simulink model "vehicle_sim"  (R2018b)
settings: Solver=VariableStepAuto  StartTime=0.0  StopTime=10.0  RelTol=1e-3
values from neighbouring files (symbols this model uses):
  delta_step = dmax/15    (= 0.0407243492132)    [vehicle_sim_main.m]
  Td_step = Tdmax/2.5    (= 353.3586)    [vehicle_sim_main.m]
  th = [m;Jz;a;b;Cf;Cr;rw;mu;Af;Al;Cx;Rr;rho]    [Parameters.m]    (also in vehicle_sim_main.m = [m;Jz;a;b;Cf;Cr;rw;mu;Tdmax;Tdmin;dmax;dmin;Af;Al;Cx;Rr;rho])
  Ts_slk = 1e-1    (= 0.1)    [vehicle_sim_main.m]
  xi0 = [X Y Ux beta psi r]'    [Vehicle_Project_Main.m]    (also in Vehicle_Project_Main_Edo.m; Vehicle_Project_Main_torque.m; initial_guess_setting.m; nonchiude.mat = [1.99964684616 -50.0000753453 20 0 -7.1628861126e-05 0])
settings Model: Creator=Lorenzo  LastModifiedBy=Lorenzo

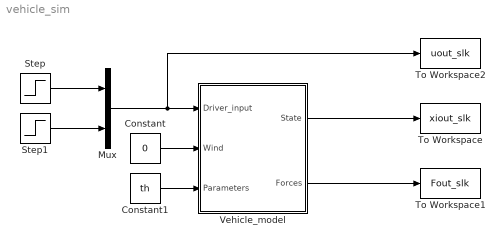
== system vehicle_sim ==
  Constant : Constant  Value=0
  Constant1 : Constant  Value=th
  Mux : Mux  Inputs=2
  Step : Step  Time=0  After=Td_step  SampleTime=0
  Step1 : Step  Time=0  After=delta_step  SampleTime=0
  To Workspace : ToWorkspace  VariableName=xiout_slk  SaveFormat=Structure With Time  SampleTime=Ts_slk
  To Workspace1 : ToWorkspace  VariableName=Fout_slk  SaveFormat=Structure With Time  SampleTime=Ts_slk
  To Workspace2 : ToWorkspace  VariableName=uout_slk  SaveFormat=Structure With Time  SampleTime=Ts_slk
  Vehicle_model : Subsystem
  wires:
  Vehicle_model/1(State) -> To Workspace/1
  Vehicle_model/2(Forces) -> To Workspace1/1
  Step/1 -> Mux/1
  Step1/1 -> Mux/2
  Mux/1 -> To Workspace2/1, Vehicle_model/1(Driver_input)
  Constant/1 -> Vehicle_model/2(Wind)
  Constant1/1 -> Vehicle_model/3(Parameters)

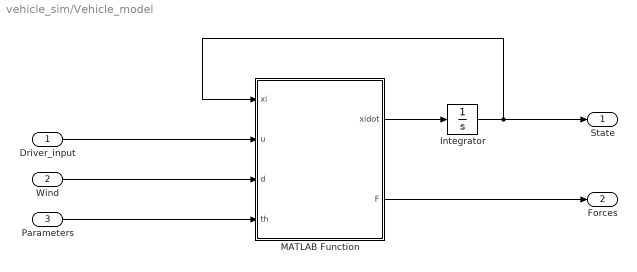
== system vehicle_sim/Vehicle_model ==
  Driver_input : Inport
  Wind : Inport  Port=2
  Parameters : Inport  Port=3
  Integrator : Integrator  InitialCondition=xi0
  MATLAB Function : MATLAB Function  TreatAsAtomicUnit=on
  State : Outport
  Forces : Outport  Port=2
  wires:
  Parameters/1 -> MATLAB Function/4(th)
  Integrator/1 -> State/1, MATLAB Function/1(xi)
  Wind/1 -> MATLAB Function/3(d)
  MATLAB Function/1(xidot) -> Integrator/1
  Driver_input/1 -> MATLAB Function/2(u)
  MATLAB Function/2(F) -> Forces/1

== matlab function vehicle_sim/Vehicle_model/MATLAB Function ==
  data: xi input; u input; xidot output; d input; th input; F output
function [xidot,F]=vehicle_model(xi,u,d,th)
% Nonlinear dynamic model of a road vehicle with six states: 2-D position,
% 2-D velocity, yaw angle and yaw rate. Nonlinear lateral tyre forces with
% Fiala model; saturation on braking and driving torque, saturation on 
% front wheel steering angle. Partial de-coupling of longitudinal and
% lateral dynamics (assume longitudinal speed varies slowly with respect to
% lateral dynamics)
%
% Inputs:   xi      (model state)
%           u       (braking/driving torque and steering angle)
%           d       (lateral wind),
%           
%           th      (model parameters)
%
% Outputs:  xi_dot  (derivative of the state with respect to time)
%           F       (longitudinal and lateral forces)

%% Read parameters, states and inputs
% Parameters
m       =       th(1,1);     % vehicle mass (kg)
Jz      =       th(2,1);     % vehicle moment of inertia (kg*m^2)
a       =       th(3,1);     % distance between center of gravity and front axle (m)
b       =       th(4,1);     % distance between center of gravity and rear axle (m)
Cf      =       th(5,1);     % front axle cornering stiffness (N/rad)
Cr      =       th(6,1);     % rear axle cornering stiffness (N/rad)
rw      =       th(7,1);     % wheel radius (m)
mu      =       th(8,1);     % road friction coefficient
Af      =       th(13,1);    % vehicle front surface (m^2)
Al      =       th(14,1);    % vehicle lateral surface (m^2)
Cx      =       th(15,1);    % vehicle front aerodynamic drag coefficient
Rr      =       th(16,1);    % rolling resistance coefficient(N*s/m)
rho     =       th(17,1);    % air density (kg/m^3)

% States
X       =       xi(1,1);    % inertial X position (m)
Y       =       xi(2,1);    % inertial Y position (m)
Ux      =       xi(3,1);    % body x velocity (m/s)
beta    =       xi(4,1);    % sideslip angle (rad)
psi     =       xi(5,1);    % yaw angle (rad)
r       =       xi(6,1);    % yaw rate (rad/s)

% Inputs
Td      =       u(1,1);     % driving/braking torque (N*m)
delta   =       u(2,1);     % front wheel steering angle (rad)
W       =       d(1,1);     % lateral wind speed (m/s)

%% Compute lateral and longitudinal tyre forces
Fzf     =       m*b*9.81/(a+b);             % vertical force on front axle
Fzr     =       m*a*9.81/(a+b);             % vertical force on rear axle
Uy      =       Ux*tan(beta);               % body y velocity (m/s)
alphaf  =       atan((Uy+r*a)/Ux)-delta;    % front slip angle (rad)         
zf      =       tan(alphaf);                % tangent of front slip angle
zr      =       (Uy-r*b)/Ux;                % tangent of rear slip angle
Fyf     =       min(mu*Fzf,max(-mu*Fzf,-Cf*zf+Cf^2*abs(zf)*zf/(3*mu*Fzf)-Cf^3/(27*mu^2*Fzf^2)*zf^3));   % Front lateral force (N)
Fyr     =       min(mu*Fzr,max(-mu*Fzr,-Cr*zr+Cr^2*abs(zr)*zr/(3*mu*Fzr)-Cr^3/(27*mu^2*Fzr^2)*zr^3));   % Rear lateral force (N)
Fx      =       Td/rw;                      % Longitudinal driving/braking force (N)
Fr      =       Ux*Rr;                      % Rolling resistance (N)
Fxd     =       0.5*rho*Cx*Af*Ux^2;         % Front aerodynamic resistance (N)
Fyd     =       0.5*rho*Al*W^2;             % Lateral force due to wind (N)
F       =       [Fyf;Fyr;Fx;Fr;Fxd;Fyd];

% Model equations
xidot       =   zeros(6,1);
xidot(1,1)  =   Ux*cos(psi)-Uy*sin(psi);
xidot(2,1)  =   Ux*sin(psi)+Uy*cos(psi);
xidot(3,1)  =   (Fx-Fyf*sin(delta)-Fr-Fxd)/m;
xidot(4,1)  =   (Fyf*cos(delta)+Fyr+Fyd)/(m*Ux)-r;
xidot(5,1)  =   r;
xidot(6,1)  =   (a*Fyf*cos(delta)-b*Fyr)/Jz;
